simulink model "Wood_Berry_ma"  (R2020b)
settings: Solver=ode45  StartTime=0.0  StopTime=100  MaxStep=1e-3  MinStep=1e-4  RelTol=1e-3
undefined symbols (not defined in the file or in its folder): thetad1, thetad2
libraries: cstblocks x6
settings Model: Creator=Gustavo Caldas  LastModifiedBy=Gustavo Caldas

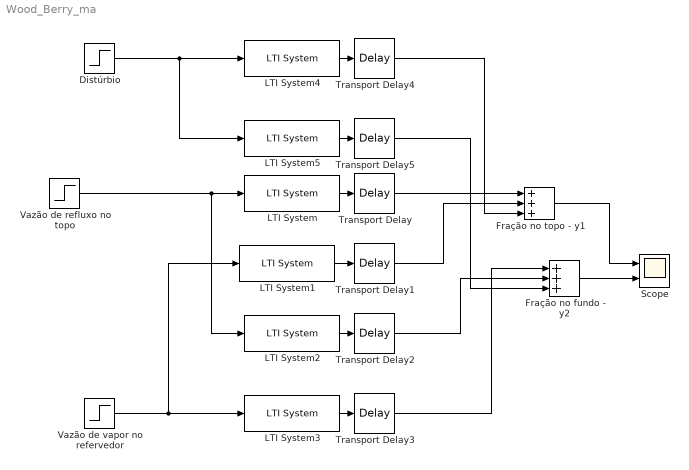
== system Wood_Berry_ma ==
  Distúrbio : Step  Time=0  After=0  SampleTime=0
  Fração no fundo - y2 : Sum  Inputs=+++
  Fração no topo - y1 : Sum  Inputs=+++
  LTI System : cstblocks/LTI System  sys=tf11  IC=[]
  LTI System1 : cstblocks/LTI System  sys=tf12  IC=[]
  LTI System2 : cstblocks/LTI System  sys=tf21  IC=[]
  LTI System3 : cstblocks/LTI System  sys=tf22  IC=[]
  LTI System4 : cstblocks/LTI System  sys=tfd1  IC=[]
  LTI System5 : cstblocks/LTI System  sys=tfd2  IC=[]
  Scope : Scope  NumInputPorts=2
  Transport Delay : TransportDelay
  Transport Delay1 : TransportDelay  DelayTime=3
  Transport Delay2 : TransportDelay  DelayTime=7
  Transport Delay3 : TransportDelay  DelayTime=3
  Transport Delay4 : TransportDelay  DelayTime=thetad1
  Transport Delay5 : TransportDelay  DelayTime=thetad2
  Vazão de refluxo no topo : Step  Time=0  SampleTime=0
  Vazão de vapor no refervedor : Step  Time=50  SampleTime=0
  wires:
  Vazão de refluxo no topo/1 -> LTI System2/1, LTI System/1
  LTI System/1 -> Transport Delay/1
  Fração no topo - y1/1 -> Scope/1
  Fração no fundo - y2/1 -> Scope/2
  LTI System3/1 -> Transport Delay3/1
  Vazão de vapor no refervedor/1 -> LTI System1/1, LTI System3/1
  LTI System1/1 -> Transport Delay1/1
  LTI System2/1 -> Transport Delay2/1
  Transport Delay/1 -> Fração no topo - y1/1
  Transport Delay1/1 -> Fração no topo - y1/2
  Transport Delay2/1 -> Fração no fundo - y2/2
  Transport Delay3/1 -> Fração no fundo - y2/1
  LTI System4/1 -> Transport Delay4/1
  LTI System5/1 -> Transport Delay5/1
  Distúrbio/1 -> LTI System5/1, LTI System4/1
  Transport Delay4/1 -> Fração no topo - y1/3
  Transport Delay5/1 -> Fração no fundo - y2/3
